simulink subsystem "EncodersCP"  (R2023b)
settings: Solver=VariableStepAuto  StartTime=0.0  StopTime=10.0  RelTol=1e-3
libraries: arduinosensorlib x2
settings Model: Creator=Carlos  LastModifiedBy=Carlos

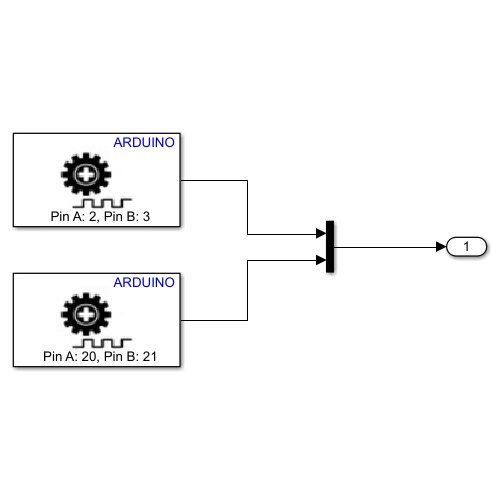
[thumbnail: Simulink's stored preview of the top-level diagram]
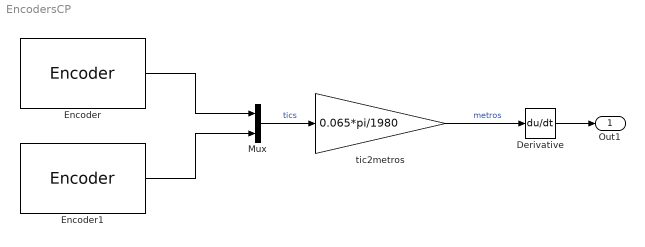
== system EncodersCP ==
  Derivative : Derivative
  Encoder : arduinosensorlib/Encoder  InputA=2  InputB=3  Mode=No reset  SampleTime=-1
  Encoder1 : arduinosensorlib/Encoder  InputA=20  InputB=21  Mode=No reset  SampleTime=-1
  Mux : Mux  Inputs=2
  tic2metros : Gain  Gain=0.065*pi/1980  OutDataTypeStr=double
  Out1 : Outport
  wires:
  Encoder/1 -> Mux/1
  Encoder1/1 -> Mux/2
  Mux/1 -> tic2metros/1  "tics"
  tic2metros/1 -> Derivative/1  "metros"
  Derivative/1 -> Out1/1
